simulink model "can_multiple_messages"  (R2024a)
settings: Solver=FixedStepDiscrete  StartTime=0.0  StopTime=inf  RelTol=1e-3
model workspace (MAT data in the model file):
  Ts = 0.01
  board_ID = 1
undefined symbols (not defined in the file): CAN_ANGLE_DEG2ICUB, canChannel, MCControlModes
libraries: canmsglib x8, canlib x2, hdlsllib x1, sldrtlib x1
settings Model: DataDictionary=amcbldc.sldd  Creator=mfussi  LastModifiedBy=mfussi
settings DebuggingCC: ParamSuppressDoubleToSinglePrecisionLossMsg=on
settings HardwareCC: ProdBitPerLong=64  ProdHWDeviceType=Intel->x86-64 (Linux 64)
settings RTWCC: Description=Simulink Desktop Real-Time  SystemTargetFile=sldrt.tlc  TemplateMakefile=sldrt.tmf  RTWCompilerOptimization=on
settings CodeAppCC: MaxIdLength=95
settings SimulinkDesktopRealTimeCC: TargetLibSuffix=_sldrt.a  TargetPreCompLibLocation=C:\Program Files\MATLAB\R2024a\toolbox\sldrt\lib\win64

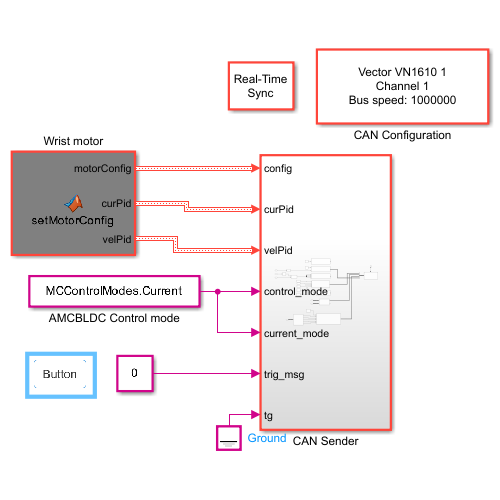
[thumbnail: Simulink's stored preview of the top-level diagram]
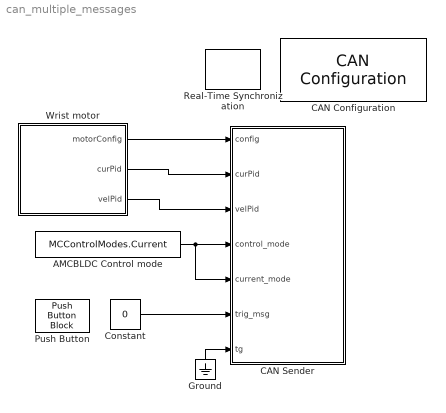
== system can_multiple_messages ==
  AMCBLDC Control mode : Constant  Value=MCControlModes.Current
  CAN Configuration : canlib/CAN Configuration  BlockHandle=12086.0011  Device=Vector VN1610 1 (Channel 1)  DeviceMenu=Vector VN1610 1 (Channel 1)  ObjConstructor=canChannel('Vector', 'VN1610 1', 1)  BusSpeed=1000000  EnableBitParameters=off  SJW=1  TSEG1=4  TSEG2=3  NSamples=1  AckMode=Normal
  CAN Sender : Subsystem
      settings: PortSchema="{\"entries\":[{\"content\":{\"sides\":[{\"content\":{},\"type\":\"ConnectorPlacement.EquallySpacedRectSide\",\"uuid\":\"bdd6ce9e-9b65-4aba-9b48-f09f8c1326bb\"},{\"content\":{\"side\":\"RIGHT\"},\"type\":\"ConnectorPlacement.EquallySpacedRectSide\",\"uuid\":\"141c9ef5-f742-47fc-b635-015c7474b58f\"},{\"content\":{\"connectorIds\":[\"In1\",\"In2\",\"In3\",\"In4\",\"In5\",\"In6\",\"In7\"],\"side\":\"TOP\"},\"type\":\"ConnectorPlacement.EquallySpacedRectSide\",\"uuid\":\"624889ac-74c5-4b05-9d21-0587daea952f\"}]},\"type\":\"ConnectorPlacement.EquallySpacedConnector\",\"uuid\":\"a748afda-e52d-41b4-a312-ee668058905d\"}],\"packageUris\":[\"http://schema.mathworks.com/mf0/Connector/R2020b\"],\"version\":\"1.0\"}"
  Constant : Constant  Value=0
  Ground : Ground
  Push Button : PushButtonBlock  OffValue=0.000000
  Real-Time Synchronization : sldrtlib/Real-Time Synchronization  SampleTime=Ts  MaxMissedTicks=inf  ShowMissedTicks=off  YieldWhenWaiting=off
  Wrist motor : MATLAB Function  TreatAsAtomicUnit=on
  wires:
  Ground/1 -> CAN Sender/1(tg)
  Wrist motor/1(motorConfig) -> CAN Sender/7(config)
  Wrist motor/2(curPid) -> CAN Sender/6(curPid)
  Wrist motor/3(velPid) -> CAN Sender/5(velPid)
  AMCBLDC Control mode/1 -> CAN Sender/3(current_mode), CAN Sender/4(control_mode)
  Constant/1 -> CAN Sender/2(trig_msg)

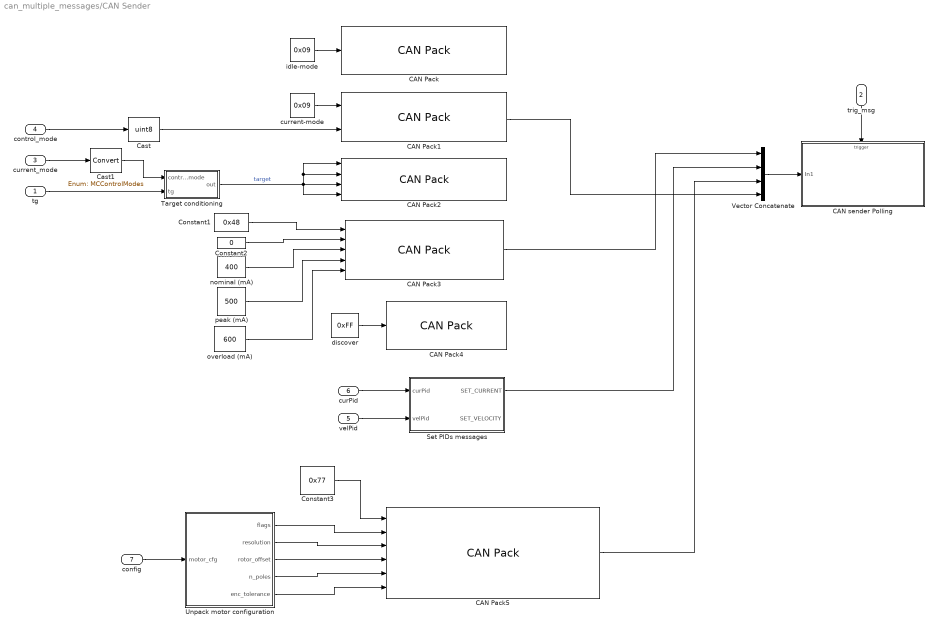
== system can_multiple_messages/CAN Sender ==
  tg : Inport
  trig_msg : Inport  Port=2
  current_mode : Inport  Port=3
  control_mode : Inport  Port=4
  velPid : Inport  Port=5
  curPid : Inport  Port=6
  config : Inport  Port=7
  CAN Pack : canmsglib/CAN Pack  MsgList=(none)  MsgName=CAN Idle  MsgIDType=Standard (11-bit identifier)  MsgIdentifier=board_ID  MsgLength=2  Remote=off  ApplyMinMax=off  BusOutput=on  SignalInfo={ 'Idle', '0', '16', 'LE', 'unsigned', 'Standard', '0', '1', '0', '-Inf', 'Inf' }
      settings: DataFormat=manually specified signals
  CAN Pack1 : canmsglib/CAN Pack  MsgList=(none)  MsgName=SET Control Mode  MsgIDType=Standard (11-bit identifier)  MsgIdentifier=board_ID  MsgLength=2  Remote=off  ApplyMinMax=off  BusOutput=on  SignalInfo={ 'CMD', '0', '8', 'LE', 'unsigned', 'Standard', '0', '1', '0', '-Inf', 'Inf'; 'CTRL', '8', '8', 'LE', 'signed', 'Standard', '0', '1', '0', '-Inf', 'Inf' }
      settings: DataFormat=manually specified signals
  CAN Pack2 : canmsglib/CAN Pack  MsgList=(none)  MsgName=CAN Target  MsgIDType=Standard (11-bit identifier)  MsgIdentifier=0x10F  MsgLength=8  Remote=off  ApplyMinMax=off  BusOutput=on  SignalInfo={ 'Target 1', '0', '16', 'LE', 'signed', 'Standard', '0', '1', '0', '-Inf', 'Inf'; 'Target 2', '16', '16', 'LE', 'signed', 'Standard', '0', '1', '0', '-Inf', 'Inf'; 'Target 3', '32', '16', 'LE', 'signed', 'Standard', '0', '1', '0', '-Inf', 'Inf'; 'Target 4', '48', '16', 'LE', 'signed', 'Standard', '0', '1', '0', '-Inf', 'Inf' }
      settings: DataFormat=manually specified signals
  CAN Pack3 : canmsglib/CAN Pack  MsgList=(none)  MsgName=CAN Limits  MsgIDType=Standard (11-bit identifier)  MsgIdentifier=board_ID  MsgLength=8  Remote=off  ApplyMinMax=off  BusOutput=on  SignalInfo={ 'CMD', '0', '8', 'LE', 'unsigned', 'Standard', '0', '1', '0', '-Inf', 'Inf'; 'X', '8', '8', 'LE', 'unsigned', 'Standard', '0', '1', '0', '-Inf', 'Inf'; 'NOMINAL', '16', '16', 'LE', 'unsigned', 'Standard', '0', '1', '0', '-Inf', 'Inf'; 'PEAK', '32', '16', 'LE', 'unsigned', 'Standard', '0', '1', '0', '-Inf', 'Inf'; 'OVERLOAD', '48', '16', 'LE', 'unsigned', 'Standard', '0', '1', '0', '-Inf', 'Inf' }
      settings: DataFormat=manually specified signals
  CAN Pack4 : canmsglib/CAN Pack  MsgList=(none)  MsgName=DISCOVER  MsgIDType=Standard (11-bit identifier)  MsgIdentifier=0x70F  MsgLength=1  Remote=off  ApplyMinMax=off  BusOutput=on  SignalInfo={}
      settings: DataFormat=raw data
  CAN Pack5 : canmsglib/CAN Pack  MsgList=(none)  MsgName=Set_Motor_Config  MsgIDType=Standard (11-bit identifier)  MsgIdentifier=board_ID  MsgLength=8  Remote=off  ApplyMinMax=off  BusOutput=on  SignalInfo={ 'CMD', '0', '8', 'LE', 'unsigned', 'Standard', '0', '1', '0', '-Inf', 'Inf'; 'FLAGS', '8', '8', 'LE', 'unsigned', 'Standard', '0', '1', '0', '-Inf', 'Inf'; 'RES_ENCODER', '16', '16', 'LE', 'signed', 'Standard', '0', '1', '0', '-Inf', 'Inf'; 'OFFSET_ENCODER', '32', '16', 'LE', 'unsigned', 'Standard', '0', '1', '0', '-Inf', 'Inf'; 'N_POLES', '48', '8', 'LE', 'unsigned', 'Standard', '0', '1', '0', '-Inf', 'Inf'; 'ENCODER_TOLERANCE', '56', '8', 'LE', 'unsigned', 'Standard', '0', '1', '0', '-Inf', 'Inf' }
      settings: DataFormat=manually specified signals
  CAN sender Polling : Subsystem
  Cast : DataTypeConversion  OutDataTypeStr=uint8  SaturateOnIntegerOverflow=off  RndMeth=Floor
  Cast1 : DataTypeConversion  OutDataTypeStr=Enum: MCControlModes  SaturateOnIntegerOverflow=off  RndMeth=Floor
  Constant1 : Constant  Value=0x48  OutDataTypeStr=Inherit: Inherit via back propagation
  Constant2 : Constant  Value=0  OutDataTypeStr=Inherit: Inherit via back propagation
  Constant3 : Constant  Value=0x77  OutDataTypeStr=Inherit: Inherit via back propagation
  Set PIDs messages : Subsystem
  Target conditioning : Subsystem
  Unpack motor configuration : MATLAB Function  TreatAsAtomicUnit=on
  Vector Concatenate : Concatenate  NumInputs=4
  current-mode : Constant  Value=0x09  OutDataTypeStr=Inherit: Inherit via back propagation
  discover : Constant  Value=0xFF
  idle-mode : Constant  Value=0x09  OutDataTypeStr=Inherit: Inherit via back propagation
  nominal (mA) : Constant  Value=400  OutDataTypeStr=Inherit: Inherit via back propagation
  overload (mA) : Constant  Value=600  OutDataTypeStr=Inherit: Inherit via back propagation
  peak (mA) : Constant  Value=500  OutDataTypeStr=Inherit: Inherit via back propagation
  wires:
  idle-mode/1 -> CAN Pack/1
  current-mode/1 -> CAN Pack1/1
  Constant1/1 -> CAN Pack3/1
  discover/1 -> CAN Pack4/1
  trig_msg/1 -> CAN sender Polling/Trigger
  Constant2/1 -> CAN Pack3/2
  nominal (mA)/1 -> CAN Pack3/3
  peak (mA)/1 -> CAN Pack3/4
  overload (mA)/1 -> CAN Pack3/5
  Vector Concatenate/1 -> CAN sender Polling/1(In1)
  control_mode/1 -> Cast/1
  Constant3/1 -> CAN Pack5/1
  velPid/1 -> Set PIDs messages/2(velPid)
  config/1 -> Unpack motor configuration/1(motor_cfg)
  curPid/1 -> Set PIDs messages/1(curPid)
  Unpack motor configuration/1(flags) -> CAN Pack5/2
  Unpack motor configuration/2(resolution) -> CAN Pack5/3
  Unpack motor configuration/3(rotor_offset) -> CAN Pack5/4
  Unpack motor configuration/4(n_poles) -> CAN Pack5/5
  Unpack motor configuration/5(enc_tolerance) -> CAN Pack5/6
  tg/1 -> Target conditioning/2(tg)
  Target conditioning/1(out) -> CAN Pack2/4, CAN Pack2/1, CAN Pack2/2, CAN Pack2/3  "target"
  Cast/1 -> CAN Pack1/2
  Cast1/1 -> Target conditioning/1(control_mode)
  current_mode/1 -> Cast1/1
  CAN Pack3/1 -> Vector Concatenate/1
  Set PIDs messages/1(SET_CURRENT) -> Vector Concatenate/2
  CAN Pack5/1 -> Vector Concatenate/3
  CAN Pack1/1 -> Vector Concatenate/4

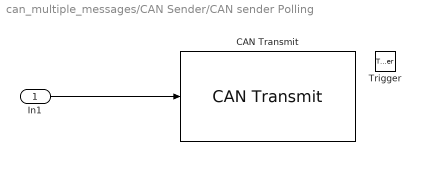
== system can_multiple_messages/CAN Sender/CAN sender Polling ==
  In1 : Inport
  Trigger : TriggerPort  VariantControl=(inherit)  PortDimensions=1
  CAN Transmit : canlib/CAN Transmit  BlockHandle=12349.0013  Device=Vector VN1610 1 (Channel 1)  DeviceMenu=Vector VN1610 1 (Channel 1)  ObjConstructor=canChannel('Vector', 'VN1610 1', 1)  EnableEventTransmit=off  EnablePeriodicTransmit=off  MessagePeriod=1.000
  wires:
  In1/1 -> CAN Transmit/1

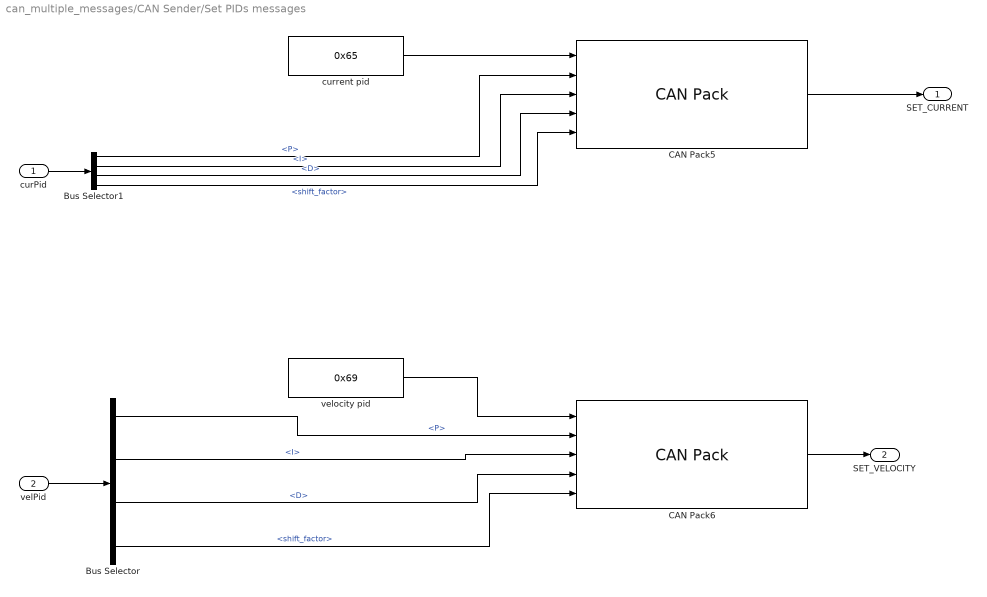
== system can_multiple_messages/CAN Sender/Set PIDs messages ==
  curPid : Inport
  velPid : Inport  Port=2
  Bus Selector : BusSelector  OutputSignals=P,I,D,shift_factor
  Bus Selector1 : BusSelector  OutputSignals=P,I,D,shift_factor
  CAN Pack5 : canmsglib/CAN Pack  MsgList=(none)  MsgName=SET_CURRENT_PID  MsgIDType=Standard (11-bit identifier)  MsgIdentifier=board_ID  MsgLength=8  Remote=off  ApplyMinMax=off  BusOutput=on  SignalInfo={ 'CMD', '0', '8', 'LE', 'unsigned', 'Standard', '0', '1', '0', '-Inf', 'Inf'; 'Kp', '8', '16', 'LE', 'signed', 'Standard', '0', '1', '0', '-Inf', 'Inf'; 'Ki', '24', '16', 'LE', 'signed', 'Standard', '0', '1', '0', '-Inf', 'Inf'; 'Kd', '40', '16', 'LE', 'signed', 'Standard', '0', '1', '0', '-Inf', 'Inf'; 'shift', '56', '8', 'LE', 'unsigned', 'Standard', '0', '1', '0', '-Inf', 'Inf' }
      settings: DataFormat=manually specified signals
  CAN Pack6 : canmsglib/CAN Pack  MsgList=(none)  MsgName=SET_VELOCITY_PID  MsgIDType=Standard (11-bit identifier)  MsgIdentifier=board_ID  MsgLength=8  Remote=off  ApplyMinMax=off  BusOutput=on  SignalInfo={ 'CMD', '0', '8', 'LE', 'unsigned', 'Standard', '0', '1', '0', '-Inf', 'Inf'; 'Kp', '8', '16', 'LE', 'signed', 'Standard', '0', '1', '0', '-Inf', 'Inf'; 'Ki', '24', '16', 'LE', 'signed', 'Standard', '0', '1', '0', '-Inf', 'Inf'; 'Kd', '40', '16', 'LE', 'signed', 'Standard', '0', '1', '0', '-Inf', 'Inf'; 'shift', '56', '8', 'LE', 'unsigned', 'Standard', '0', '1', '0', '-Inf', 'Inf' }
      settings: DataFormat=manually specified signals
  current pid : Constant  Value=0x65  OutDataTypeStr=int16
  velocity pid : Constant  Value=0x69  OutDataTypeStr=int16
  SET_CURRENT : Outport
  SET_VELOCITY : Outport  Port=2
  wires:
  Bus Selector/4 -> CAN Pack6/5  "<shift_factor>"
  Bus Selector/1 -> CAN Pack6/2  "<P>"
  Bus Selector1/4 -> CAN Pack5/5  "<shift_factor>"
  Bus Selector1/1 -> CAN Pack5/2  "<P>"
  Bus Selector/3 -> CAN Pack6/4  "<D>"
  Bus Selector/2 -> CAN Pack6/3  "<I>"
  Bus Selector1/2 -> CAN Pack5/3  "<I>"
  current pid/1 -> CAN Pack5/1
  velocity pid/1 -> CAN Pack6/1
  CAN Pack5/1 -> SET_CURRENT/1
  CAN Pack6/1 -> SET_VELOCITY/1
  velPid/1 -> Bus Selector/1
  curPid/1 -> Bus Selector1/1
  Bus Selector1/3 -> CAN Pack5/4  "<D>"

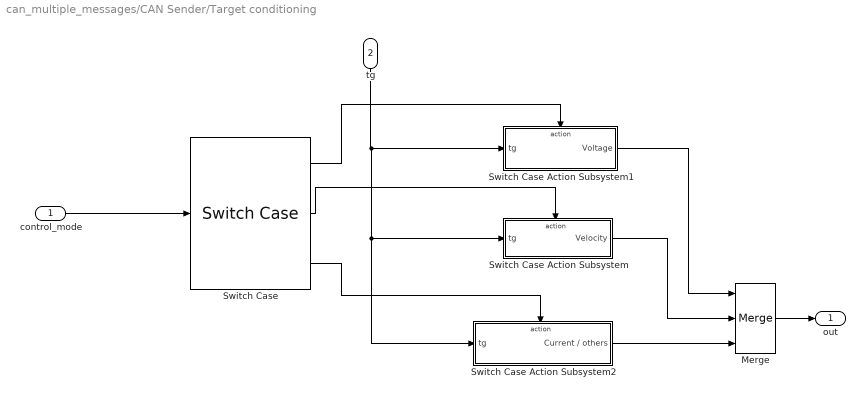
== system can_multiple_messages/CAN Sender/Target conditioning ==
  control_mode : Inport
  tg : Inport  Port=2
  Merge : Merge  Inputs=3
  Switch Case : SwitchCase  CaseConditions={MCControlModes.OpenLoop, MCControlModes.SpeedVoltage}
  Switch Case Action Subsystem : Subsystem  TreatAsAtomicUnit=on
  Switch Case Action Subsystem1 : Subsystem  TreatAsAtomicUnit=on
  Switch Case Action Subsystem2 : Subsystem  TreatAsAtomicUnit=on
  out : Outport
  wires:
  tg/1 -> Switch Case Action Subsystem2/1(tg), Switch Case Action Subsystem/1(tg), Switch Case Action Subsystem1/1(tg)
  Switch Case/1 -> Switch Case Action Subsystem1/Action
  Switch Case/2 -> Switch Case Action Subsystem/Action
  Switch Case/3 -> Switch Case Action Subsystem2/Action
  Merge/1 -> out/1
  control_mode/1 -> Switch Case/1
  Switch Case Action Subsystem1/1(Voltage) -> Merge/1
  Switch Case Action Subsystem/1(Velocity) -> Merge/2
  Switch Case Action Subsystem2/1(Current / others) -> Merge/3

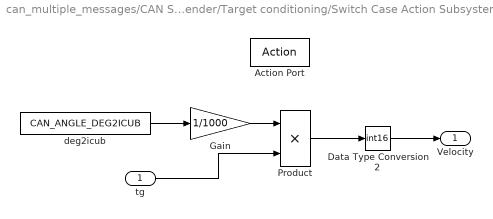
== system can_multiple_messages/CAN Sender/Target conditioning/Switch Case Action Subsystem ==
  tg : Inport
  Action Port : ActionPort  ActionPortLabel=case [ SpeedVoltage ]:
  Data Type Conversion2 : DataTypeConversion  OutDataTypeStr=int16  SaturateOnIntegerOverflow=off  RndMeth=Floor
  Gain : Gain  Gain=1/1000
  Product : Product
  deg2icub : Constant  Value=CAN_ANGLE_DEG2ICUB  OutDataTypeStr=single
  Velocity : Outport
  wires:
  tg/1 -> Product/2
  Gain/1 -> Product/1
  deg2icub/1 -> Gain/1
  Product/1 -> Data Type Conversion2/1
  Data Type Conversion2/1 -> Velocity/1

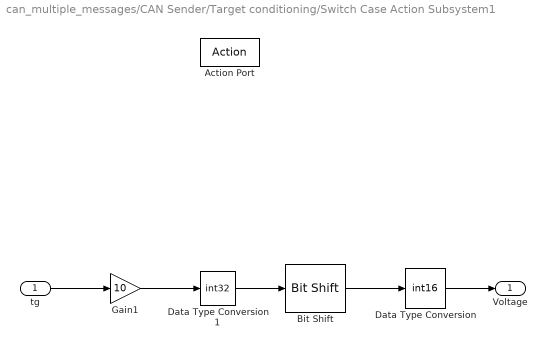
== system can_multiple_messages/CAN Sender/Target conditioning/Switch Case Action Subsystem1 ==
  tg : Inport
  Action Port : ActionPort  ActionPortLabel=case [ OpenLoop ]:
  Bit Shift : hdlsllib/Logic and Bit Operations/Bit Shift  mode=Shift Left Logical  N=5
  Data Type Conversion : DataTypeConversion  OutDataTypeStr=int16  SaturateOnIntegerOverflow=off  RndMeth=Floor
  Data Type Conversion1 : DataTypeConversion  OutDataTypeStr=int32  SaturateOnIntegerOverflow=off  RndMeth=Floor
  Gain1 : Gain  Gain=10
  Voltage : Outport
  wires:
  Bit Shift/1 -> Data Type Conversion/1
  Gain1/1 -> Data Type Conversion1/1
  tg/1 -> Gain1/1
  Data Type Conversion/1 -> Voltage/1
  Data Type Conversion1/1 -> Bit Shift/1

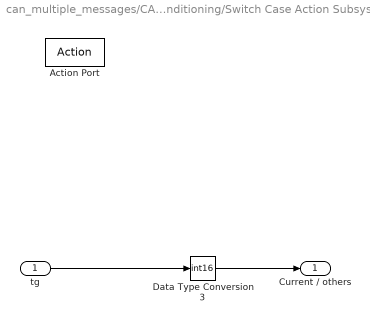
== system can_multiple_messages/CAN Sender/Target conditioning/Switch Case Action Subsystem2 ==
  tg : Inport
  Action Port : ActionPort  ActionPortLabel=default:
  Data Type Conversion3 : DataTypeConversion  OutDataTypeStr=int16  SaturateOnIntegerOverflow=off  RndMeth=Floor
  Current / others : Outport
  wires:
  tg/1 -> Data Type Conversion3/1
  Data Type Conversion3/1 -> Current / others/1

== matlab function can_multiple_messages/Wrist motor ==
  data: motorConfig output Bus: MotorConfigurationExternal; curPid output Bus: PID; velPid output Bus: PID
function [motorConfig, curPid, velPid] = setMotorConfig()


motorConfig.enable_verbosity = false;
motorConfig.has_hall_sens = true;
motorConfig.has_quadrature_encoder = false;
motorConfig.has_speed_quadrature_encoder = false;
motorConfig.has_torque_sens = false;
motorConfig.encoder_tolerance = uint8(0);
motorConfig.pole_pairs = uint8(7);
motorConfig.rotor_encoder_resolution = int16(0); % set to 0 to use only hall sensors
motorConfig.rotor_index_offset = int16(0);
motorConfig.use_index = false;


% motorConfig.Kbemf = single(0);
% motorConfig.Rphase = single(0);
% motorConfig.Imin = single(-1e3);
% motorConfig.Imax = single(1e3);
% motorConfig.Vmax = single(44);
% motorConfig.resistance = single(25.9);
% motorConfig.inductance = single(271);
% motorConfig.thermal_resistance = single(56);
% motorConfig.thermal_time_constant = single(270);

% Hall offset and BC phases swap is not available as a CAN message
% The parameters need to be changed in rtw_motor_config.c
swap_bc = 1;

% ---------------------------------

curPid.type = ControlModes.Current;
curPid.OutMax = single(100);
curPid.OutMin = single(-100);
% curPid.P = single(0.271);
% curPid.I = single(25900);
curPid.P = single(2);
curPid.I = single(500);
curPid.D = single(0);
curPid.N = single(100);
curPid.I0 = single(0);
curPid.D0 = single(0);
% curPid.shift_factor = uint8(6);
curPid.shift_factor = uint8(0);

velPid.type = ControlModes.Velocity;
velPid.OutMax = single(1000);
velPid.OutMin = single(-1000);
velPid.P = single(-20);
velPid.I = single(-20);
velPid.D = single(0);
velPid.N = single(100);
velPid.I0 = single(0);
velPid.D0 = single(0);
velPid.shift_factor = uint8(10);

== matlab function can_multiple_messages/CAN Sender/Unpack motor configuration ==
  data: flags output; resolution output; rotor_offset output; n_poles output; motor_cfg input; enc_tolerance output
function [flags, resolution,rotor_offset, n_poles, enc_tolerance] = unpack_cfg(motor_cfg)

    flags = uint8(motor_cfg.has_quadrature_encoder); 
    flags = bitor(flags, bitshift(uint8(motor_cfg.has_hall_sens), 1));
    resolution = motor_cfg.rotor_encoder_resolution;
    rotor_offset = motor_cfg.rotor_index_offset;
    n_poles = motor_cfg.pole_pairs * 2;
    enc_tolerance = motor_cfg.encoder_tolerance;

end
